simulink model "Fixed_Wing_Aircraft_Sim"  (R2020b)
settings: Solver=ode15s  StartTime=0.0  StopTime=10000  MinStep=1e-200  RelTol=1e-3
InitFcn:
  | parameters
undefined symbols (not defined in the file or in its folder): drawAircraft, plotmavstatevariables
settings Model: Creator=Pravin  LastModifiedBy=pravi
settings DataIOCC: ReturnWorkspaceOutputs=off
settings DebuggingCC: ArithmeticOperatorsInVariantConditions=warning
settings SFSimCC: SimUseLocalCustomCode=off  CustomCodeUndefinedFunction=UseInterfaceOnly
settings RTWCC: RTWUseLocalCustomCode=off
settings CodeAppCC: StateflowObjectComments=on

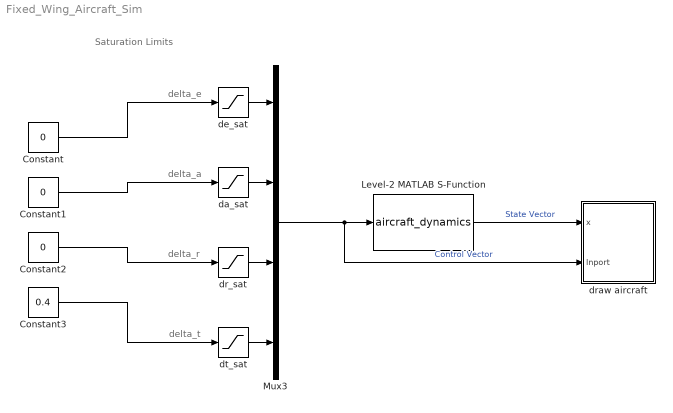
== system Fixed_Wing_Aircraft_Sim ==
  note: Saturation Limits
  note: delta_t
  note: delta_a
  note: delta_r
  note: delta_e
  Constant : Constant  Value=0
  Constant1 : Constant  Value=0
  Constant2 : Constant  Value=0
  Constant3 : Constant  Value=0.4
  Level-2 MATLAB S-Function : M-S-Function  FunctionName=aircraft_dynamics  Parameters=P
  Mux3 : Mux
  da_sat : Saturate  UpperLimit=50  LowerLimit=-50
  de_sat : Saturate  UpperLimit=50  LowerLimit=-50
  dr_sat : Saturate  UpperLimit=50  LowerLimit=-50
  draw aircraft : Subsystem
  dt_sat : Saturate  UpperLimit=1  LowerLimit=0
  wires:
  Level-2 MATLAB S-Function/1 -> draw aircraft/1(x)  "State Vector"
  Mux3/1 -> draw aircraft/2(Inport), Level-2 MATLAB S-Function/1  "Control Vector"
  dt_sat/1 -> Mux3/4
  de_sat/1 -> Mux3/1
  Constant3/1 -> dt_sat/1
  Constant2/1 -> dr_sat/1
  Constant1/1 -> da_sat/1
  da_sat/1 -> Mux3/2
  dr_sat/1 -> Mux3/3
  Constant/1 -> de_sat/1

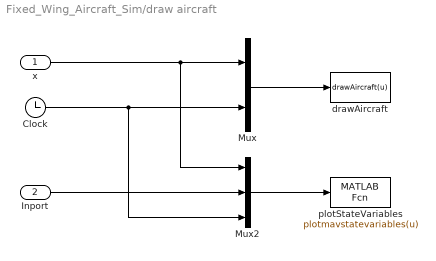
== system Fixed_Wing_Aircraft_Sim/draw aircraft ==
  x : Inport
  Inport : Inport  Port=2
  Clock : Clock
  Mux : Mux  Inputs=2
  Mux2 : Mux  Inputs=3
  drawAircraft : MATLABFcn  MATLABFcn=drawAircraft(u)  OutputDimensions=0  SampleTime=0.1
  plotStateVariables : MATLABFcn  MATLABFcn=plotmavstatevariables(u)  OutputDimensions=0  SampleTime=0.1
  wires:
  Clock/1 -> Mux2/3, Mux/2
  x/1 -> Mux2/1, Mux/1
  Mux/1 -> drawAircraft/1
  Mux2/1 -> plotStateVariables/1
  Inport/1 -> Mux2/2
